simulink model "WiperSystemControl"  (R2024b)
settings: Solver=VariableStepAuto  StartTime=0.0  StopTime=10.0  MaxStep=1e-3  RelTol=1e-3
undefined symbols (not defined in the file or in its folder): WiperSystemModes
libraries: simulink x1
settings Model: Creator=MOHAMED  LastModifiedBy=MOHAMED

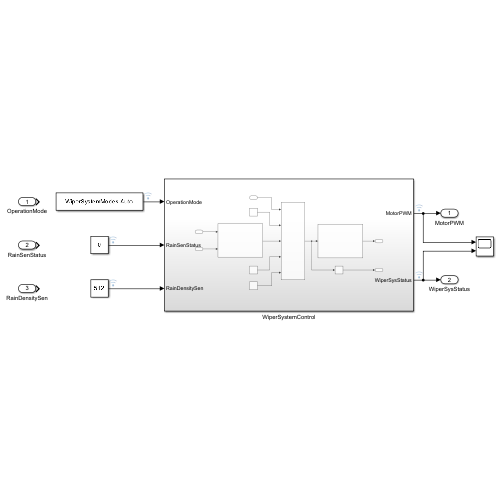
[thumbnail: Simulink's stored preview of the top-level diagram]
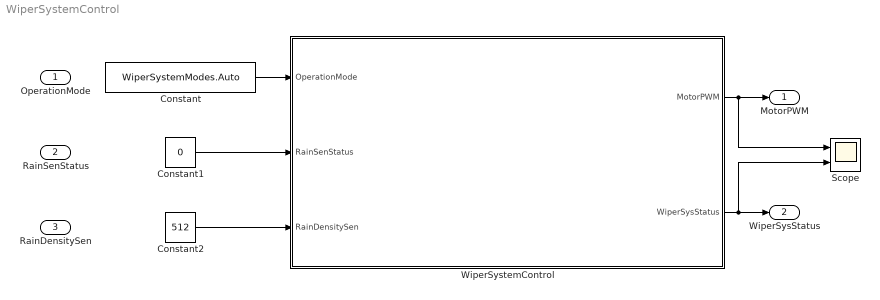
== system WiperSystemControl ==
  OperationMode : Inport
  RainSenStatus : Inport  Port=2
  RainDensitySen : Inport  Port=3
  Constant : Constant  Value=WiperSystemModes.Auto
  Constant1 : Constant  Value=0
  Constant2 : Constant  Value=512
  Scope : Scope  NumInputPorts=2
  WiperSystemControl : Subsystem
  MotorPWM : Outport
  WiperSysStatus : Outport  Port=2
  wires:
  WiperSystemControl/1(MotorPWM) -> Scope/1, MotorPWM/1
  WiperSystemControl/2(WiperSysStatus) -> Scope/2, WiperSysStatus/1
  Constant/1 -> WiperSystemControl/1(OperationMode)
  Constant1/1 -> WiperSystemControl/2(RainSenStatus)
  Constant2/1 -> WiperSystemControl/3(RainDensitySen)

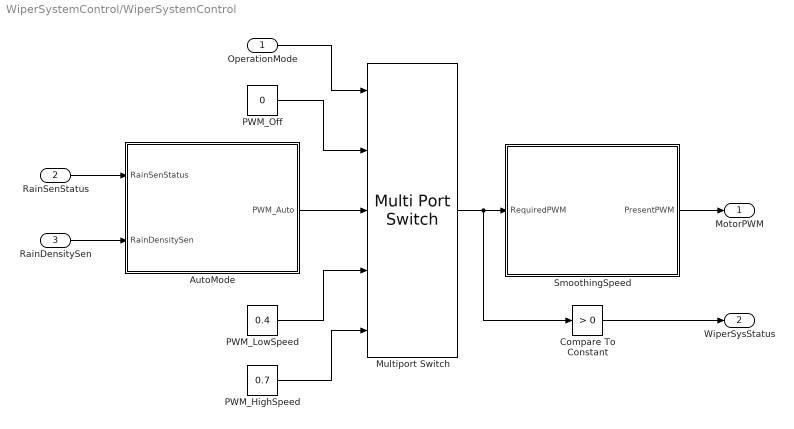
== system WiperSystemControl/WiperSystemControl ==
  OperationMode : Inport
  RainSenStatus : Inport  Port=2
  RainDensitySen : Inport  Port=3
  AutoMode : Subsystem  TreatAsAtomicUnit=on
  Compare To Constant : simulink/Logic and Bit Operations/Compare To Constant  relop=>  const=0  OutDataTypeStr=boolean
  Multiport Switch : MultiPortSwitch  DataPortOrder=Specify indices  Inputs=4  DataPortIndices={WiperSystemModes.Off, WiperSystemModes.Auto, WiperSystemModes.LowSpeed, WiperSystemModes.HighSpeed}  SaturateOnIntegerOverflow=off  InputSameDT=off
  PWM_HighSpeed : Constant  Value=0.7
  PWM_LowSpeed : Constant  Value=0.4
  PWM_Off : Constant  Value=0
  SmoothingSpeed : Subsystem
  MotorPWM : Outport
  WiperSysStatus : Outport  Port=2
  wires:
  RainDensitySen/1 -> AutoMode/2(RainDensitySen)
  RainSenStatus/1 -> AutoMode/1(RainSenStatus)
  Multiport Switch/1 -> SmoothingSpeed/1(RequiredPWM), Compare To Constant/1
  OperationMode/1 -> Multiport Switch/1
  PWM_Off/1 -> Multiport Switch/2
  PWM_LowSpeed/1 -> Multiport Switch/4
  AutoMode/1(PWM_Auto) -> Multiport Switch/3
  PWM_HighSpeed/1 -> Multiport Switch/5
  SmoothingSpeed/1(PresentPWM) -> MotorPWM/1
  Compare To Constant/1 -> WiperSysStatus/1

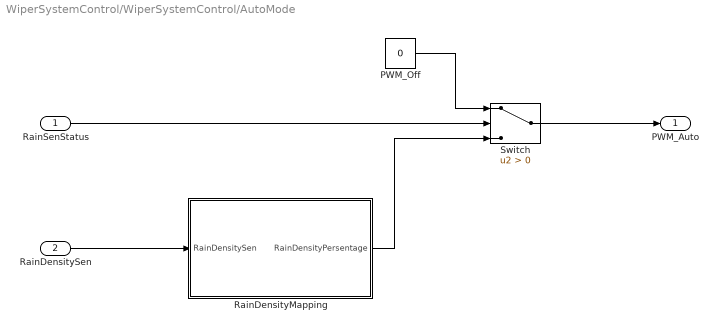
== system WiperSystemControl/WiperSystemControl/AutoMode ==
  RainSenStatus : Inport
  RainDensitySen : Inport  Port=2
  PWM_Off : Constant  Value=0
  RainDensityMapping : Subsystem
  Switch : Switch  Criteria=u2 > Threshold  SaturateOnIntegerOverflow=off  InputSameDT=off
  PWM_Auto : Outport
  wires:
  RainSenStatus/1 -> Switch/2
  RainDensityMapping/1(RainDensityPersentage) -> Switch/3
  RainDensitySen/1 -> RainDensityMapping/1(RainDensitySen)
  PWM_Off/1 -> Switch/1
  Switch/1 -> PWM_Auto/1

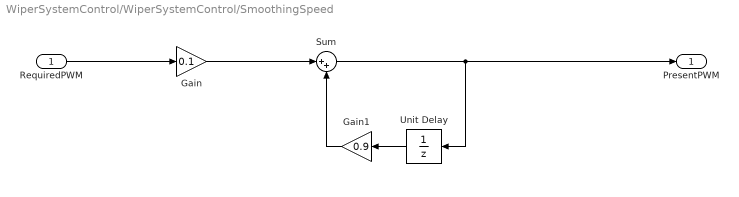
== system WiperSystemControl/WiperSystemControl/SmoothingSpeed ==
  RequiredPWM : Inport
  Gain : Gain  Gain=0.1
  Gain1 : Gain  Gain=0.9
  Sum : Sum  Inputs=|++
  Unit Delay : UnitDelay  SampleTime=-1  HasFrameUpgradeWarning=on
  PresentPWM : Outport
  wires:
  RequiredPWM/1 -> Gain/1
  Gain/1 -> Sum/1
  Sum/1 -> Unit Delay/1, PresentPWM/1
  Unit Delay/1 -> Gain1/1
  Gain1/1 -> Sum/2

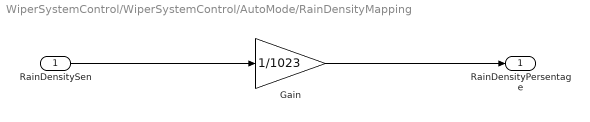
== system WiperSystemControl/WiperSystemControl/AutoMode/RainDensityMapping ==
  RainDensitySen : Inport
  Gain : Gain  Gain=1/1023
  RainDensityPersentage : Outport
  wires:
  RainDensitySen/1 -> Gain/1
  Gain/1 -> RainDensityPersentage/1
